simulink model "aocs_attitude_plant"  (R2025a)
settings: Solver=ode45  StartTime=0  StopTime=200  RelTol=1e-09  AbsTol=1e-10
undefined symbols (not defined in the file): AOCS_Config
settings Model: Creator=juliankazmierski  LastModifiedBy=juliankazmierski

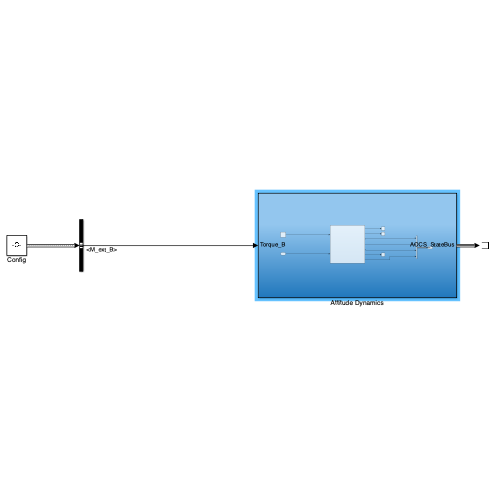
[thumbnail: Simulink's stored preview of the top-level diagram]
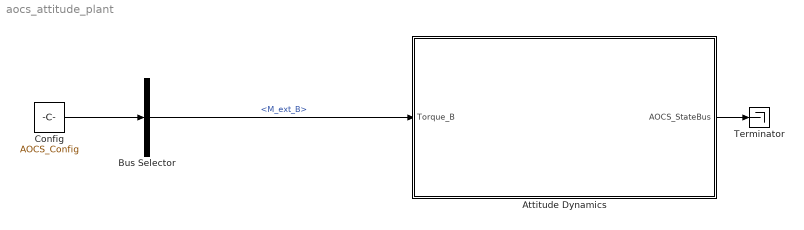
== system aocs_attitude_plant ==
  Attitude Dynamics : Subsystem
  Bus Selector : BusSelector  OutputSignals=M_ext_B
  Config : Constant  Value=AOCS_Config  OutDataTypeStr=Bus: AOCS_ConfigBus
  Terminator : Terminator
  wires:
  Bus Selector/1 -> Attitude Dynamics/1(Torque_B)  "<M_ext_B>"
  Config/1 -> Bus Selector/1
  Attitude Dynamics/1(AOCS_StateBus) -> Terminator/1

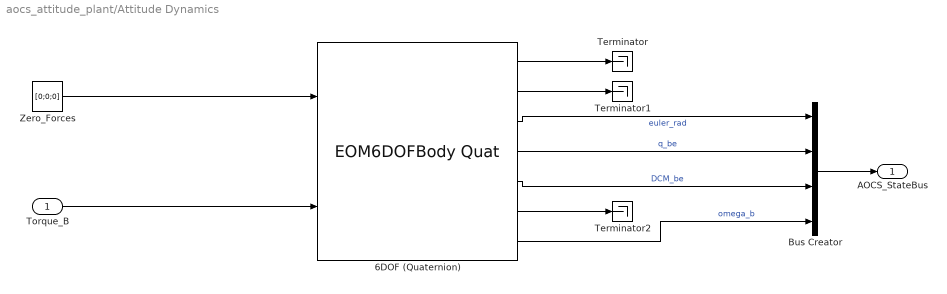
== system aocs_attitude_plant/Attitude Dynamics ==
  Torque_B : Inport
  6DOF (Quaternion) : EOM6DOFBodyQuat  eul_0=AOCS_Config.euler_BI_0_rad  pm_0=AOCS_Config.omega_BI_B_0  mass_0=3.71  inertia=AOCS_Config.I_B
  Bus Creator : BusCreator  Inputs=4
  Terminator : Terminator
  Terminator1 : Terminator
  Terminator2 : Terminator
  Zero_Forces : Constant  Value=[0;0;0]
  AOCS_StateBus : Outport  OutDataTypeStr=Bus: AOCS_StateBus
  wires:
  Torque_B/1 -> 6DOF (Quaternion)/2
  Zero_Forces/1 -> 6DOF (Quaternion)/1
  6DOF (Quaternion)/1 -> Terminator/1
  6DOF (Quaternion)/2 -> Terminator1/1
  6DOF (Quaternion)/6 -> Terminator2/1
  6DOF (Quaternion)/3 -> Bus Creator/1  "euler_rad"
  6DOF (Quaternion)/5 -> Bus Creator/3  "DCM_be"
  6DOF (Quaternion)/7 -> Bus Creator/4  "omega_b"
  Bus Creator/1 -> AOCS_StateBus/1
  6DOF (Quaternion)/4 -> Bus Creator/2  "q_be"
